simulink model "Output_Sliding_Mode_Control"  (R2021b)
settings: Solver=VariableStepAuto  StartTime=tspan(1)  StopTime=tspan(2)  RelTol=1e-9
undefined symbols (not defined in the file): BL_gain, K_switch, lambda_1_num, lambda_2_num, r_sim, Tmax, x_0
settings Model: Creator=domin  LastModifiedBy=domin
settings SolverCC: AlgebraicLoopSolver=TrustRegion
settings DebuggingCC: SFMachineParentedDataDiag=warning

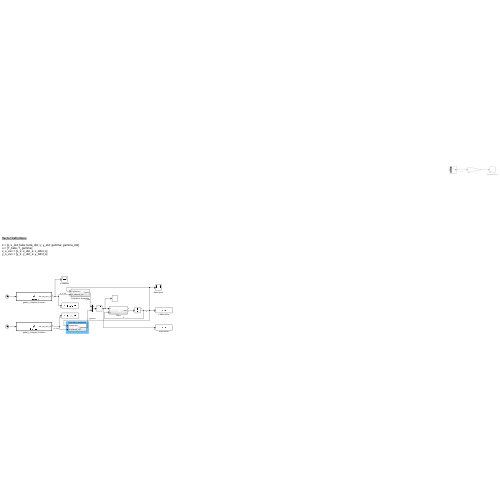
[thumbnail: Simulink's stored preview of the top-level diagram]
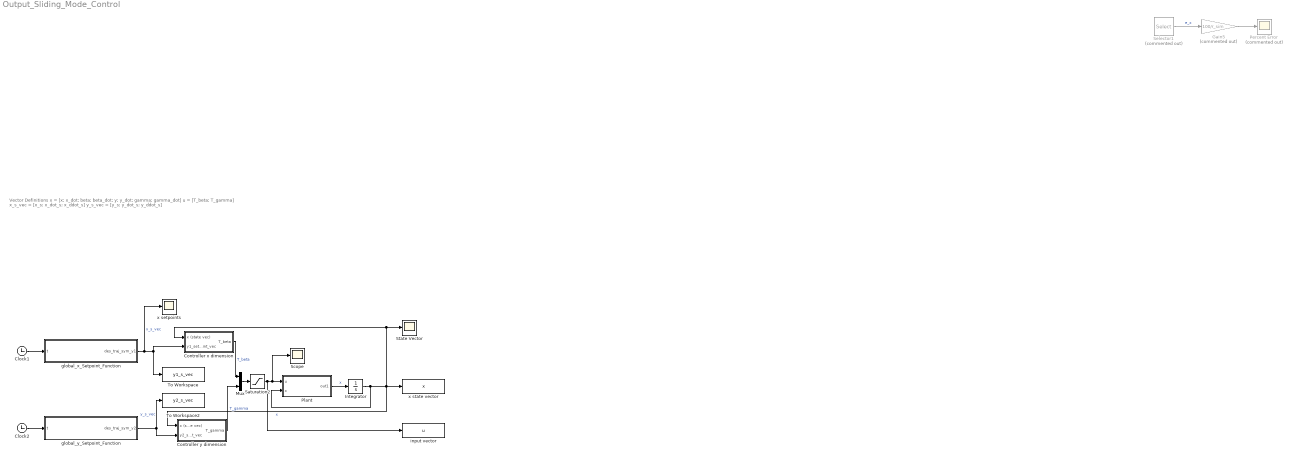
== system Output_Sliding_Mode_Control ==
  note: Vector Definitions
      |
      | x = [x; x_dot; beta; beta_dot; y; y_dot; gamma; gamma_dot]
      | u = [T_beta; T_gamma]
      | x_s_vec = [x_s; x_dot_s; x_ddot_s]
      | y_s_vec = [y_s; y_dot_s; y_ddot_s]
  Clock1 : Clock
  Clock2 : Clock
  Controller x dimension : Subsystem
  Controller y dimension : Subsystem
  Gain5 : Gain  Commented=on  Gain=100/r_sim
  Integrator : Integrator  InitialCondition=x_0
  Mux : Mux  Inputs=2
  Percent Error : Scope  Commented=on
  Plant : Subsystem
  Saturation2 : Saturate  UpperLimit=Tmax  LowerLimit=-Tmax  ZeroCross=off
  Scope : Scope
  Selector1 : Selector  Commented=on  InputPortWidth=5  IndexOptions=Index vector (dialog)  Indices=[1]  OutputSizes=1
  State Vector : Scope
  To Workspace : ToWorkspace  VariableName=y1_s_vec  SampleTime=-1
  To Workspace2 : ToWorkspace  VariableName=y2_s_vec  SampleTime=-1
  global_x_Setpoint_Function : MATLAB Function  TreatAsAtomicUnit=on
  global_y_Setpoint_Function : MATLAB Function  TreatAsAtomicUnit=on
  input vector : ToWorkspace  VariableName=u  SampleTime=-1
  x setpoints : Scope
  x state vector : ToWorkspace  VariableName=x  SampleTime=-1
  wires:
  global_x_Setpoint_Function/1(des_traj_sym_y1) -> x setpoints/1, To Workspace/1, Controller x dimension/2(y1_setpoint_vec)  "x_s_vec"
  Integrator/1 -> Plant/2(x), x state vector/1, Controller y dimension/1(x (state vec)), Controller x dimension/1(x (state vec)), State Vector/1  "x"
  Plant/1(out1) -> Integrator/1  "x"
  Clock1/1 -> global_x_Setpoint_Function/1(t)
  Gain5/1 -> Percent Error/1
  Selector1/1 -> Gain5/1  "e_x"
  Clock2/1 -> global_y_Setpoint_Function/1(t)
  Controller x dimension/1(T_beta) -> Mux/1  "T_beta"
  Controller y dimension/1(T_gamma) -> Mux/2  "T_gamma"
  global_y_Setpoint_Function/1(des_traj_sym_y2) -> Controller y dimension/2(y2_setpoint_vec), To Workspace2/1  "y_s_vec"
  Mux/1 -> Saturation2/1
  Saturation2/1 -> Scope/1, Plant/1(u), input vector/1

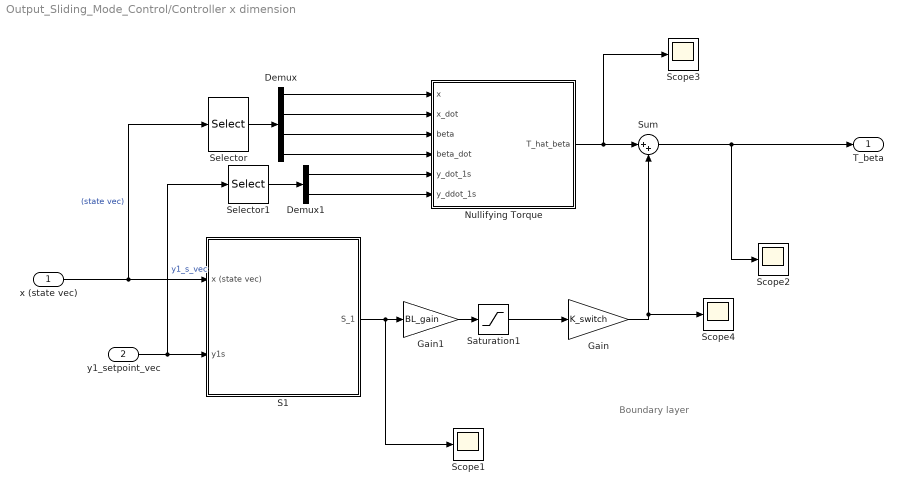
== system Output_Sliding_Mode_Control/Controller x dimension ==
  note: Boundary layer
  x (state vec) : Inport
  y1_setpoint_vec : Inport  Port=2
  Demux : Demux
  Demux1 : Demux  Outputs=2
  Gain : Gain  Gain=K_switch
  Gain1 : Gain  Gain=BL_gain
  Nullifying Torque : MATLAB Function  TreatAsAtomicUnit=on
  S1 : Subsystem
  Saturation1 : Saturate  UpperLimit=1  LowerLimit=-1
  Scope{1..4} (4 alike) : Scope
  Selector : Selector  InputPortWidth=8  IndexOptions=Index vector (dialog)  Indices=[1:4]  OutputSizes=1
  Selector1 : Selector  InputPortWidth=3  IndexOptions=Index vector (dialog)  Indices=[2 3]  OutputSizes=1
  Sum : Sum  Inputs=|++
  T_beta : Outport
  wires:
  Sum/1 -> Scope2/1, T_beta/1
  x (state vec)/1 -> Selector/1, S1/1(x (state vec))  "(state vec)"
  y1_setpoint_vec/1 -> Selector1/1, S1/2(y1s)  "y1_s_vec"
  S1/1(S_1) -> Gain1/1, Scope1/1
  Selector/1 -> Demux/1
  Demux/1 -> Nullifying Torque/1(x)
  Demux/2 -> Nullifying Torque/2(x_dot)
  Demux/3 -> Nullifying Torque/3(beta)
  Demux/4 -> Nullifying Torque/4(beta_dot)
  Selector1/1 -> Demux1/1
  Demux1/1 -> Nullifying Torque/5(y_dot_1s)
  Demux1/2 -> Nullifying Torque/6(y_ddot_1s)
  Nullifying Torque/1(T_hat_beta) -> Scope3/1, Sum/1
  Saturation1/1 -> Gain/1
  Gain/1 -> Sum/2, Scope4/1
  Gain1/1 -> Saturation1/1

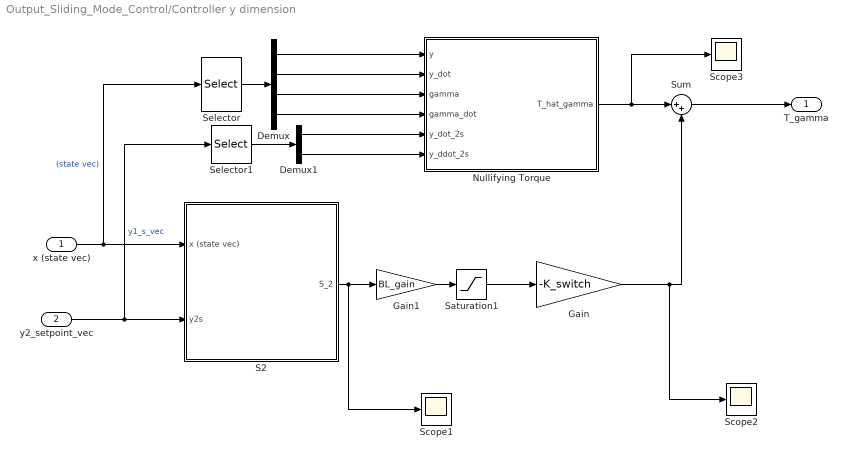
== system Output_Sliding_Mode_Control/Controller y dimension ==
  x (state vec) : Inport
  y2_setpoint_vec : Inport  Port=2
  Demux : Demux
  Demux1 : Demux  Outputs=2
  Gain : Gain  Gain=-K_switch
  Gain1 : Gain  Gain=BL_gain
  Nullifying Torque : MATLAB Function  TreatAsAtomicUnit=on
  S2 : Subsystem
  Saturation1 : Saturate  UpperLimit=1  LowerLimit=-1
  Scope1 : Scope
  Scope2 : Scope
  Scope3 : Scope
  Selector : Selector  InputPortWidth=8  IndexOptions=Index vector (dialog)  Indices=[5:8]  OutputSizes=1
  Selector1 : Selector  InputPortWidth=3  IndexOptions=Index vector (dialog)  Indices=[2 3]  OutputSizes=1
  Sum : Sum  Inputs=|++
  T_gamma : Outport
  wires:
  S2/1(S_2) -> Scope1/1, Gain1/1
  Gain/1 -> Sum/2, Scope2/1
  Saturation1/1 -> Gain/1
  Demux/2 -> Nullifying Torque/2(y_dot)
  Nullifying Torque/1(T_hat_gamma) -> Scope3/1, Sum/1
  Demux1/1 -> Nullifying Torque/5(y_dot_2s)
  Selector/1 -> Demux/1
  Demux/3 -> Nullifying Torque/3(gamma)
  Demux/4 -> Nullifying Torque/4(gamma_dot)
  Selector1/1 -> Demux1/1
  Demux1/2 -> Nullifying Torque/6(y_ddot_2s)
  x (state vec)/1 -> S2/1(x (state vec)), Selector/1  "(state vec)"
  Demux/1 -> Nullifying Torque/1(y)
  y2_setpoint_vec/1 -> S2/2(y2s), Selector1/1  "y1_s_vec"
  Sum/1 -> T_gamma/1
  Gain1/1 -> Saturation1/1

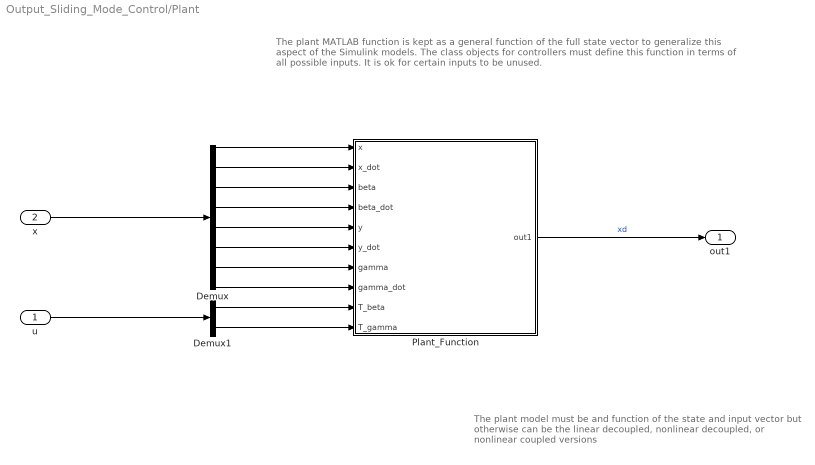
== system Output_Sliding_Mode_Control/Plant ==
  note: The plant MATLAB function is kept as a general function of the full state vector
      | to generalize this aspect of the Simulink models. The class objects for controllers must define this function in terms of all possible inputs. It is ok for certain inputs to be unused.
  note: The plant model must be and function of the state and input vector
      |  but otherwise can be the linear decoupled, nonlinear decoupled,
      | or nonlinear coupled versions
  u : Inport
  x : Inport  Port=2
  Demux : Demux  Outputs=8
  Demux1 : Demux  Outputs=2
  Plant_Function : MATLAB Function  TreatAsAtomicUnit=on
  out1 : Outport
  wires:
  Demux1/1 -> Plant_Function/9(T_beta)
  Demux1/2 -> Plant_Function/10(T_gamma)
  Demux/5 -> Plant_Function/5(y)
  Demux/8 -> Plant_Function/8(gamma_dot)
  Demux/7 -> Plant_Function/7(gamma)
  Demux/1 -> Plant_Function/1(x)
  Demux/3 -> Plant_Function/3(beta)
  Demux/4 -> Plant_Function/4(beta_dot)
  Demux/2 -> Plant_Function/2(x_dot)
  Demux/6 -> Plant_Function/6(y_dot)
  x/1 -> Demux/1
  Plant_Function/1(out1) -> out1/1  "xd"
  u/1 -> Demux1/1

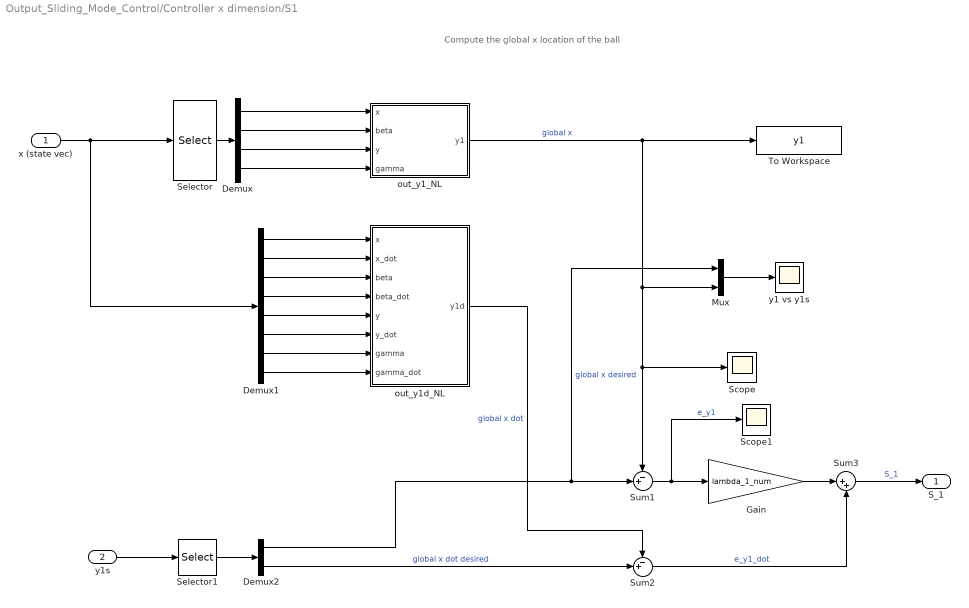
== system Output_Sliding_Mode_Control/Controller x dimension/S1 ==
  note: Compute the global x location of the ball
  x (state vec) : Inport
  y1s : Inport  Port=2
  Demux : Demux
  Demux1 : Demux  Outputs=8
  Demux2 : Demux  Outputs=2
  Gain : Gain  Gain=lambda_1_num
  Mux : Mux  Inputs=2
  Scope : Scope
  Scope1 : Scope
  Selector : Selector  InputPortWidth=8  IndexOptions=Index vector (dialog)  Indices=[1 3 5 7]  OutputSizes=1
  Selector1 : Selector  InputPortWidth=3  IndexOptions=Index vector (dialog)  Indices=[1 2]  OutputSizes=1
  Sum1 : Sum  Inputs=-+|
  Sum2 : Sum  Inputs=-+|
  Sum3 : Sum  Inputs=|++
  To Workspace : ToWorkspace  VariableName=y1  SampleTime=-1
  out_y1_NL : MATLAB Function  TreatAsAtomicUnit=on
  out_y1d_NL : MATLAB Function  TreatAsAtomicUnit=on
  y1 vs y1s : Scope
  S_1 : Outport
  wires:
  Demux/4 -> out_y1_NL/4(gamma)
  Sum3/1 -> S_1/1  "S_1"
  Selector/1 -> Demux/1
  Demux1/5 -> out_y1d_NL/5(y)
  Demux1/1 -> out_y1d_NL/1(x)
  Demux1/4 -> out_y1d_NL/4(beta_dot)
  Demux/2 -> out_y1_NL/2(beta)
  Sum1/1 -> Scope1/1, Gain/1  "e_y1"
  Sum2/1 -> Sum3/2  "e_y1_dot"
  x (state vec)/1 -> Demux1/1, Selector/1
  Gain/1 -> Sum3/1
  Demux/1 -> out_y1_NL/1(x)
  Demux/3 -> out_y1_NL/3(y)
  Demux1/2 -> out_y1d_NL/2(x_dot)
  Demux1/6 -> out_y1d_NL/6(y_dot)
  Demux1/8 -> out_y1d_NL/8(gamma_dot)
  out_y1_NL/1(y1) -> Mux/2, Scope/1, Sum1/1, To Workspace/1  "global x"
  Demux1/7 -> out_y1d_NL/7(gamma)
  Demux2/1 -> Mux/1, Sum1/2  "global x desired"
  Demux1/3 -> out_y1d_NL/3(beta)
  Demux2/2 -> Sum2/2  "global x dot desired"
  y1s/1 -> Selector1/1
  out_y1d_NL/1(y1d) -> Sum2/1  "global x dot"
  Selector1/1 -> Demux2/1
  Mux/1 -> y1 vs y1s/1

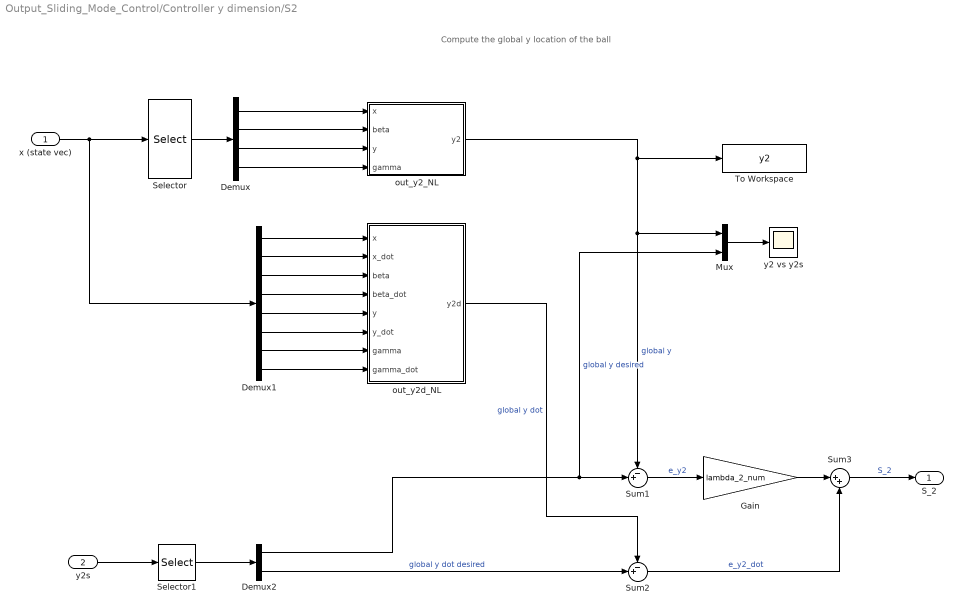
== system Output_Sliding_Mode_Control/Controller y dimension/S2 ==
  note: Compute the global y location of the ball
  x (state vec) : Inport
  y2s : Inport  Port=2
  Demux : Demux
  Demux1 : Demux  Outputs=8
  Demux2 : Demux  Outputs=2
  Gain : Gain  Gain=lambda_2_num
  Mux : Mux  Inputs=2
  Selector : Selector  InputPortWidth=8  IndexOptions=Index vector (dialog)  Indices=[1 3 5 7]  OutputSizes=1
  Selector1 : Selector  InputPortWidth=3  IndexOptions=Index vector (dialog)  Indices=[1 2]  OutputSizes=1
  Sum1 : Sum  Inputs=-+|
  Sum2 : Sum  Inputs=-+|
  Sum3 : Sum  Inputs=|++
  To Workspace : ToWorkspace  VariableName=y2  SampleTime=-1
  out_y2_NL : MATLAB Function  TreatAsAtomicUnit=on
  out_y2d_NL : MATLAB Function  TreatAsAtomicUnit=on
  y2 vs y2s : Scope
  S_2 : Outport
  wires:
  Demux/4 -> out_y2_NL/4(gamma)
  Sum3/1 -> S_2/1  "S_2"
  Selector/1 -> Demux/1
  Demux1/5 -> out_y2d_NL/5(y)
  Demux1/1 -> out_y2d_NL/1(x)
  Demux1/4 -> out_y2d_NL/4(beta_dot)
  Demux/2 -> out_y2_NL/2(beta)
  Sum1/1 -> Gain/1  "e_y2"
  Sum2/1 -> Sum3/2  "e_y2_dot"
  x (state vec)/1 -> Selector/1, Demux1/1
  Gain/1 -> Sum3/1
  Demux/1 -> out_y2_NL/1(x)
  Demux/3 -> out_y2_NL/3(y)
  Demux1/2 -> out_y2d_NL/2(x_dot)
  Demux1/6 -> out_y2d_NL/6(y_dot)
  Demux1/8 -> out_y2d_NL/8(gamma_dot)
  out_y2_NL/1(y2) -> To Workspace/1, Mux/1, Sum1/1  "global y"
  Demux1/7 -> out_y2d_NL/7(gamma)
  Demux2/1 -> Mux/2, Sum1/2  "global y desired"
  Demux1/3 -> out_y2d_NL/3(beta)
  Demux2/2 -> Sum2/2  "global y dot desired"
  y2s/1 -> Selector1/1
  out_y2d_NL/1(y2d) -> Sum2/1  "global y dot"
  Selector1/1 -> Demux2/1
  Mux/1 -> y2 vs y2s/1

== matlab function Output_Sliding_Mode_Control/Controller x dimension/S1/out_y1d_NL ==
  data: x input; y1d output; x_dot input; beta input; beta_dot input; y input; y_dot input; gamma input; gamma_dot input
function y1d = y1d(x,x_dot,beta,beta_dot,y,y_dot,gamma,gamma_dot)
%#codegen

%    This function was generated by the Symbolic Math Toolbox version 9.0.
%    20-Nov-2021 16:05:35

y1d = x_dot+beta_dot.*cos(gamma).*6.05e-2+beta_dot.*y.*sin(gamma);

== matlab function Output_Sliding_Mode_Control/Plant/Plant_Function ==
  data: x input; out1 output size=8; x_dot input; beta input; beta_dot input; y input; y_dot input; gamma input; gamma_dot input; T_beta input; T_gamma input
function out1 = xdot(x,x_dot,beta,beta_dot,y,y_dot,gamma,gamma_dot,T_beta,T_gamma)
%#codegen

%    This function was generated by the Symbolic Math Toolbox version 9.0.
%    20-Nov-2021 16:05:36

t2 = cos(beta);
t3 = cos(gamma);
t4 = sin(beta);
t5 = sin(gamma);
t6 = beta_dot.^2;
t7 = gamma_dot.^2;
t8 = x.^2;
t9 = y.^2;
t10 = t8.*(2.1e+1./1.0e+2);
t11 = t9.*(2.1e+1./1.0e+2);
t12 = t10+1.82492e-2;
t13 = t11+1.82492e-2;
t14 = 1.0./t12;
t15 = 1.0./t13;
mt1 = [x_dot,T_beta.*t14.*(-3.235e-1)+t14.*(t4.*7.3199277e-2+t4.*t8.*1.4715-t2.*x.*9.520605e-2+t6.*x.*1.34836525e-2+t6.*x.^3.*(3.0./2.0e+1)+beta_dot.*x.*x_dot.*1.941e-2),beta_dot,T_beta.*t14.*7.0+t14.*(t4.*1.183086+t2.*x.*2.0601-t6.*x.*9.705e-3-beta_dot.*x.*x_dot.*(2.1e+1./5.0e+1)),y_dot];
mt2 = [T_gamma.*t15.*3.235e-1-t15.*(t5.*7.3199277e-2+t5.*t9.*1.4715+t3.*y.*9.520605e-2-t7.*y.*1.34836525e-2-t7.*y.^3.*(3.0./2.0e+1)+gamma_dot.*y.*y_dot.*1.941e-2),gamma_dot,T_gamma.*t15.*7.0+t15.*(t5.*1.183086-t3.*y.*2.0601+t7.*y.*9.705e-3-gamma_dot.*y.*y_dot.*(2.1e+1./5.0e+1))];
out1 = reshape([mt1,mt2],8,1);

== matlab function Output_Sliding_Mode_Control/global_x_Setpoint_Function ==
  data: t input; des_traj_sym_y1 output
function des_traj_sym_y1 = y1_setpoint(t)
%#codegen

%    This function was generated by the Symbolic Math Toolbox version 9.0.
%    20-Nov-2021 16:05:36

t2 = t./4.0;
t4 = t.*pi.*(2.0./1.5e+1);
t3 = -t2;
t6 = cos(t4);
t7 = sin(t4);
t5 = exp(t3);
t8 = t5-1.0;
des_traj_sym_y1 = [t7.*t8.*(-1.0./1.0e+1);(t5.*t7)./4.0e+1-(t6.*t8.*pi)./7.5e+1;t5.*t7.*(-1.0./1.6e+2)+(t5.*t6.*pi)./1.5e+2+t7.*t8.*pi.^2.*1.777777777777778e-3];

== matlab function Output_Sliding_Mode_Control/global_y_Setpoint_Function ==
  data: t input; des_traj_sym_y2 output
function des_traj_sym_y2 = y2_setpoint(t)
%#codegen

%    This function was generated by the Symbolic Math Toolbox version 9.0.
%    20-Nov-2021 16:05:36

t2 = t./4.0;
t4 = t.*pi.*(2.0./1.5e+1);
t3 = -t2;
t6 = cos(t4);
t7 = sin(t4);
t5 = exp(t3);
t9 = t6.^2;
t10 = t7.^2;
t8 = t5-1.0;
des_traj_sym_y2 = [t6.*t7.*t8.*(-1.0./1.0e+1);t8.*t9.*pi.*(-1.0./7.5e+1)+(t8.*t10.*pi)./7.5e+1+(t5.*t6.*t7)./4.0e+1;(t5.*t9.*pi)./1.5e+2-(t5.*t10.*pi)./1.5e+2-(t5.*t6.*t7)./1.6e+2+t6.*t7.*t8.*pi.^2.*7.111111111111111e-3];

== matlab function Output_Sliding_Mode_Control/Controller y dimension/S2/out_y2_NL ==
  data: x input; y2 output; beta input; y input; gamma input
function y2 = y2(x,beta,y,gamma)
%#codegen

%    This function was generated by the Symbolic Math Toolbox version 9.0.
%    20-Nov-2021 16:05:36

y2 = sin(gamma).*(-6.05e-2)+y.*cos(gamma);

== matlab function Output_Sliding_Mode_Control/Controller x dimension/S1/out_y1_NL ==
  data: x input; y1 output; beta input; y input; gamma input
function y1 = y1(x,beta,y,gamma)
%#codegen

%    This function was generated by the Symbolic Math Toolbox version 9.0.
%    20-Nov-2021 16:05:35

t2 = sin(beta);
y1 = x.*cos(beta)+t2.*cos(gamma).*6.05e-2+t2.*y.*sin(gamma);

== matlab function Output_Sliding_Mode_Control/Controller y dimension/S2/out_y2d_NL ==
  data: x input; y2d output; x_dot input; beta input; beta_dot input; y input; y_dot input; gamma input; gamma_dot input
function y2d = y2d(x,x_dot,beta,beta_dot,y,y_dot,gamma,gamma_dot)
%#codegen

%    This function was generated by the Symbolic Math Toolbox version 9.0.
%    20-Nov-2021 16:05:36

y2d = gamma_dot.*(-6.05e-2)+y_dot-beta_dot.*x.*sin(gamma);

== matlab function Output_Sliding_Mode_Control/Controller x dimension/Nullifying Torque ==
  data: x input; T_hat_beta output; x_dot input; beta input; beta_dot input; y_dot_1s input; y_ddot_1s input
function T_hat_beta = T_hat_beta(x,x_dot,beta,beta_dot,y_dot_1s,y_ddot_1s)
%#codegen

%    This function was generated by the Symbolic Math Toolbox version 9.0.
%    20-Nov-2021 16:05:35

t2 = sin(beta);
t3 = beta_dot.^2;
t4 = x.^2;
t5 = t4.*(2.1e+1./1.0e+2);
t6 = t5+1.82492e-2;
t7 = 1.0./t6;
T_hat_beta = -(t4.*(2.1e+1./1.0e+1)+1.82492e-1).*(beta_dot.*2.016666666666667e-2+x_dot./3.0-y_dot_1s./3.0-y_ddot_1s+t2.*t7.*1.4477598e-1-t3.*x+t7.*x.*cos(beta).*2.943e-2+t3.*t7.*x.^3.*(3.0./2.0e+1)+t2.*t4.*t7.*1.4715+t3.*t7.*x.*1.28965e-2-beta_dot.*t7.*x.*x_dot.*(3.0./5.0e+2));

== matlab function Output_Sliding_Mode_Control/Controller y dimension/Nullifying Torque ==
  data: y input; T_hat_gamma output; y_dot input; gamma input; gamma_dot input; y_dot_2s input; y_ddot_2s input
function T_hat_gamma = T_hat_gamma(y,y_dot,gamma,gamma_dot,y_dot_2s,y_ddot_2s)
%#codegen

%    This function was generated by the Symbolic Math Toolbox version 9.0.
%    20-Nov-2021 16:05:36

t2 = sin(gamma);
t3 = gamma_dot.^2;
t4 = y.^2;
t5 = t4.*(2.1e+1./1.0e+2);
t6 = t5+1.82492e-2;
t7 = 1.0./t6;
T_hat_gamma = -(t4.*(2.1e+1./1.0e+1)+1.82492e-1).*(gamma_dot.*2.016666666666667e-2-y_dot./3.0+y_dot_2s./3.0+y_ddot_2s+t2.*t7.*1.4477598e-1+t3.*y-t7.*y.*cos(gamma).*2.943e-2-t3.*t7.*y.^3.*(3.0./2.0e+1)+t2.*t4.*t7.*1.4715-t3.*t7.*y.*1.28965e-2-gamma_dot.*t7.*y.*y_dot.*(3.0./5.0e+2));
